simulink model "qnetpendulum"  (R2022b)
settings: Solver=VariableStepAuto  StartTime=0.0  StopTime=10.0  RelTol=1e-3
InitFcn:
  | J_eq = 1.843e-6;
  | m = 0.0270;
  | r = 0.0826;
  | K_g = 1;
  | J_m = 1.80e-4;
  | n_g = 1;
  | n_m = 0.69;
  | L = 0.0955;
  | g = 9.9;
  | K_t = 0.0334;
  | R = 8.7;
  | 
  | a = J_eq + m * r ^ 2 + n_g * K_g ^ 2 * J_m;
  | b = m * L * r;
  | c = (4/3) * m * L ^ 2;
  | d = m * g * L;
  | e = 2.718;
  | f = (n_m * n_g * K_t * K_g) / R;
settings Model: Creator=Zonularity  LastModifiedBy=Zonularity

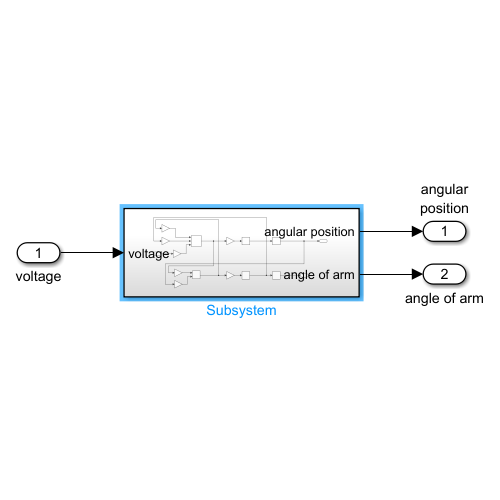
[thumbnail: Simulink's stored preview of the top-level diagram]
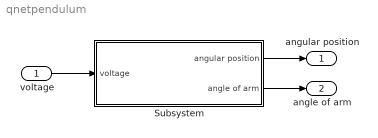
== system qnetpendulum ==
  voltage : Inport
  Subsystem : Subsystem
  angular position : Outport
  angle of arm : Outport  Port=2
  wires:
  voltage/1 -> Subsystem/1(voltage)
  Subsystem/2(angle of arm) -> angle of arm/1
  Subsystem/1(angular position) -> angular position/1

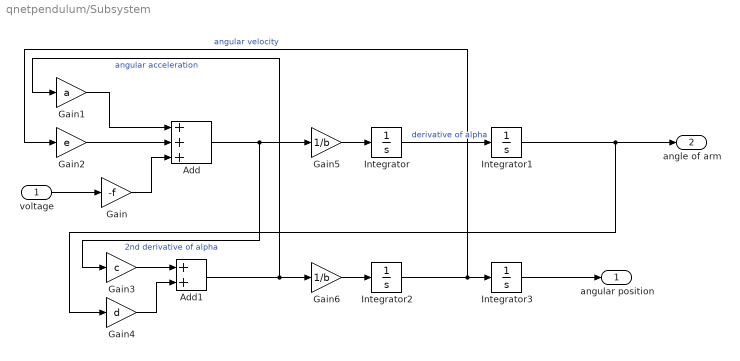
== system qnetpendulum/Subsystem ==
  voltage : Inport
  Add : Sum  Inputs=+++
  Add1 : Sum
  Gain : Gain  Gain=-f
  Gain1 : Gain  Gain=a
  Gain2 : Gain  Gain=e
  Gain3 : Gain  Gain=c
  Gain4 : Gain  Gain=d
  Gain5 : Gain  Gain=1/b
  Gain6 : Gain  Gain=1/b
  Integrator{,1..3} (4 alike) : Integrator
  angular position : Outport
  angle of arm : Outport  Port=2
  wires:
  Integrator1/1 -> angle of arm/1, Gain4/1
  Add1/1 -> Gain1/1, Gain6/1  "angular acceleration"
  Add/1 -> Gain3/1, Gain5/1  "2nd derivative of alpha"
  Integrator3/1 -> angular position/1
  Gain/1 -> Add/3
  Integrator2/1 -> Gain2/1, Integrator3/1  "angular velocity"
  Gain3/1 -> Add1/1
  Gain1/1 -> Add/1
  voltage/1 -> Gain/1
  Gain6/1 -> Integrator2/1
  Gain5/1 -> Integrator/1
  Gain2/1 -> Add/2
  Gain4/1 -> Add1/2
  Integrator/1 -> Integrator1/1  "derivative of alpha"
